simulink library "Control_Model_lib"  (R2023a)
settings: Solver=VariableStepAuto  StartTime=0.0  StopTime=10.0  RelTol=1e-3
settings Model: Creator=FIRSTMentor  LastModifiedBy=FIRSTMentor

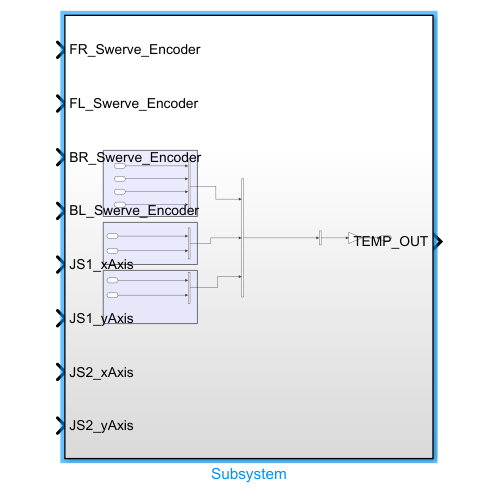
[thumbnail: Simulink's stored preview of the top-level diagram]
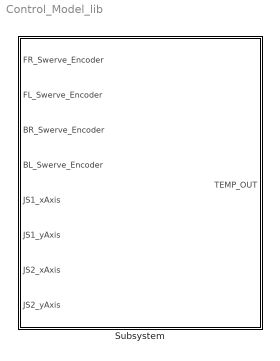
== system Control_Model_lib ==
  Subsystem : Subsystem

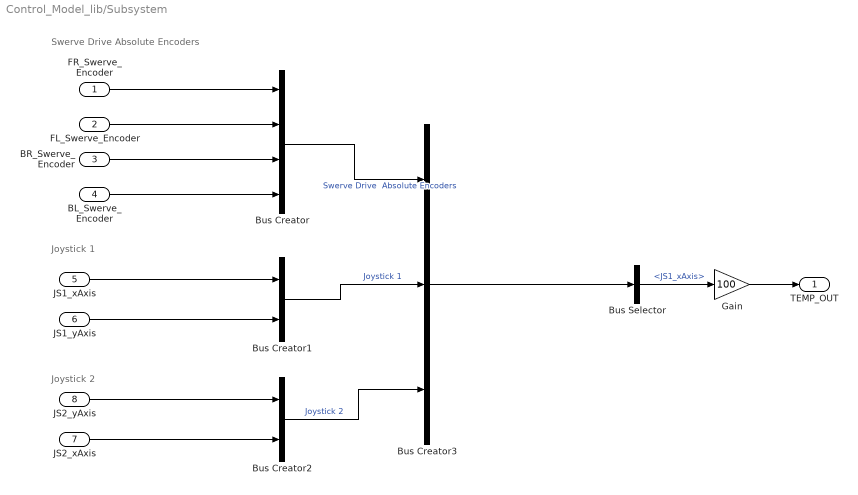
== system Control_Model_lib/Subsystem ==
  note: Swerve Drive
      | Absolute Encoders
  note: Joystick 1
  note: Joystick 2
  FR_Swerve_Encoder : Inport
  FL_Swerve_Encoder : Inport  Port=2
  BR_Swerve_Encoder : Inport  Port=3
  BL_Swerve_Encoder : Inport  Port=4
  JS1_xAxis : Inport  Port=5
  JS1_yAxis : Inport  Port=6
  JS2_xAxis : Inport  Port=7
  JS2_yAxis : Inport  Port=8
  Bus Creator : BusCreator  Inputs=4
  Bus Creator1 : BusCreator  Inputs=2
  Bus Creator2 : BusCreator  Inputs=2
  Bus Creator3 : BusCreator  Inputs=3
  Bus Selector : BusSelector  OutputSignals=Joystick 1.JS1_xAxis
  Gain : Gain  Gain=100
  TEMP_OUT : Outport
  wires:
  JS2_yAxis/1 -> Bus Creator2/1
  JS2_xAxis/1 -> Bus Creator2/2
  Bus Creator/1 -> Bus Creator3/1  "Swerve Drive  Absolute Encoders"
  BL_Swerve_Encoder/1 -> Bus Creator/4
  JS1_yAxis/1 -> Bus Creator1/2
  Bus Creator2/1 -> Bus Creator3/3  "Joystick 2"
  Gain/1 -> TEMP_OUT/1
  JS1_xAxis/1 -> Bus Creator1/1
  BR_Swerve_Encoder/1 -> Bus Creator/3
  FR_Swerve_Encoder/1 -> Bus Creator/1
  FL_Swerve_Encoder/1 -> Bus Creator/2
  Bus Selector/1 -> Gain/1  "<JS1_xAxis>"
  Bus Creator1/1 -> Bus Creator3/2  "Joystick 1"
  Bus Creator3/1 -> Bus Selector/1
